simulink model "sschdlexSwissRectifierExample"  (R2023b)
settings: Solver=FixedStepDiscrete  StartTime=0.0  StopTime=.03  RelTol=1e-3  AbsTol=1e-3
InitFcn:
  | freqMain = 50;
  | Vrms=230;
  | Vin = Vrms * sqrt(2);
  | Vout=325;
  | freqSwitch=36e3;
  | PoutMax = 7.5e3;
  | loadPercent = 50;
  | RLoad = Vout^2/(PoutMax*(loadPercent/100));
  | COut = 470e-6;
  | LDC = 305e-6;
  | LF = 85e-6;
  | CF = 4.4e-6;
libraries: fl_lib x53, nesl_utility x20, ee_lib x8, simulink x2, slpidlib x2, powerlib_meascontrol x1
settings Model: DataTypeOverride=Off  Creator=The MathWorks, Inc.  LastModifiedBy=The MathWorks, Inc.
settings SolverCC: AutoScaleAbsTol=off  AlgebraicLoopSolver=TrustRegion
settings DataIOCC: LimitDataPoints=on  MaxDataPoints=10000  SaveOutput=off  SaveTime=off  ReturnWorkspaceOutputs=off
settings OptimizationCC: BlockReduction=off  ConditionallyExecuteInputs=off  DefaultParameterBehavior=Inlined  LifeSpan=inf
settings DebuggingCC: AlgebraicLoopMsg=error  SingleTaskRateTransMsg=error  UnconnectedInputMsg=warning  UnconnectedOutputMsg=warning  UnconnectedLineMsg=warning  AllowSymbolicDim=off  PregeneratedLibrarySubsystemCodeDiagnostic=none  SFUnexpectedBacktrackingDiag=warning  SFNoUnconditionalDefaultTransitionDiag=warning  SFExecutionAtInitializationDiag=none  ArithmeticOperatorsInVariantConditions=warning
settings HardwareCC: ProdBitPerPointer=32  ProdBitPerSizeT=32  ProdBitPerPtrDiffT=32  ProdLargestAtomicFloat=None  ProdIntDivRoundTo=Undefined  ProdEndianess=Unspecified  ProdWordSize=32  ProdHWDeviceType=ASIC/FPGA->ASIC/FPGA  TargetBitPerPointer=64  TargetBitPerSizeT=64  TargetBitPerPtrDiffT=64  TargetLongLongMode=on  TargetIntDivRoundTo=Zero  TargetEndianess=LittleEndian  TargetWordSize=64  TargetHWDeviceType=Custom Processor->MATLAB Host Computer  ProdEqTarget=off
settings ModelReferenceCC: EnableRefExpFcnMdlSchedulingChecks=on
settings SFSimCC: SimUseLocalCustomCode=off
settings RTWCC: RTWUseLocalCustomCode=off
settings CodeAppCC: StateflowObjectComments=on
settings GRTTargetCC: TargetLangStandard=C89/C90 (ANSI)
settings ConfigComp: CovMetricSettings=dw  CovSaveCumulativeToWorkspaceVar=on  CovSaveSingleToWorkspaceVar=on  CovExternalEMLEnable=off  CovSFcnEnable=off
settings SimscapeCC: SimscapeLogType=all  SimscapeLogDataHistory=10000

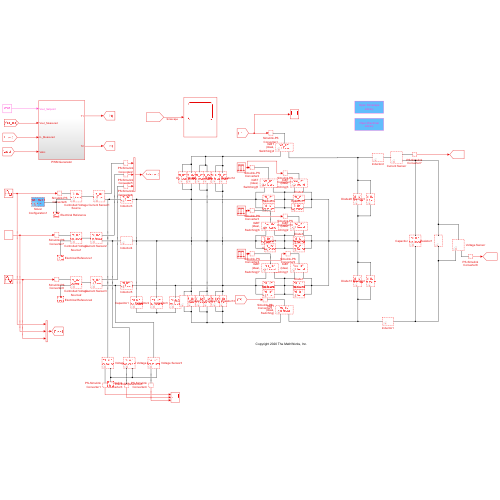
[thumbnail: Simulink's stored preview of the top-level diagram]
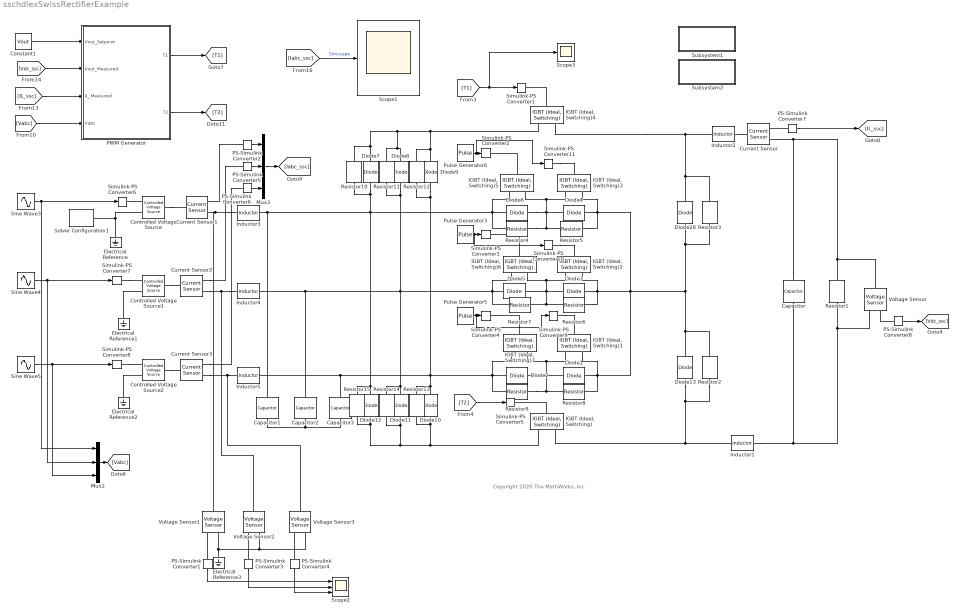
== system sschdlexSwissRectifierExample ==
  note: Copyright 2020 The MathWorks, Inc.
  Capacitor : fl_lib/Electrical/Electrical Elements/Capacitor  c=COut F  r=1e-6 Ohm  g=0 1/Ohm  i_specify=off  i_priority=None  i=0 A  i_nominal_specify=off  i_nominal_unit=A  i_nominal_value=1  v_specify=off  v_priority=None  v=0 V  v_nominal_specify=off  v_nominal_unit=V  v_nominal_value=1  vc_specify=off  vc_priority=High  vc=400 V  vc_nominal_specify=off  vc_nominal_unit=V  vc_nominal_value=1
  Capacitor1 : fl_lib/Electrical/Electrical Elements/Capacitor  c=CF F  r=1e-6 Ohm  g=0 1/Ohm  i_specify=off  i_priority=None  i=0 A  i_nominal_specify=off  i_nominal_unit=A  i_nominal_value=1  v_specify=off  v_priority=None  v=0 V  v_nominal_specify=off  v_nominal_unit=V  v_nominal_value=1  vc_specify=off  vc_priority=High  vc=0 V  vc_nominal_specify=off  vc_nominal_unit=V  vc_nominal_value=1
  Capacitor2 : fl_lib/Electrical/Electrical Elements/Capacitor  c=CF F  r=1e-6 Ohm  g=0 1/Ohm  i_specify=off  i_priority=None  i=0 A  i_nominal_specify=off  i_nominal_unit=A  i_nominal_value=1  v_specify=off  v_priority=None  v=0 V  v_nominal_specify=off  v_nominal_unit=V  v_nominal_value=1  vc_specify=off  vc_priority=High  vc=0 V  vc_nominal_specify=off  vc_nominal_unit=V  vc_nominal_value=1
  Capacitor3 : fl_lib/Electrical/Electrical Elements/Capacitor  c=CF F  r=1e-6 Ohm  g=0 1/Ohm  i_specify=off  i_priority=None  i=0 A  i_nominal_specify=off  i_nominal_unit=A  i_nominal_value=1  v_specify=off  v_priority=None  v=0 V  v_nominal_specify=off  v_nominal_unit=V  v_nominal_value=1  vc_specify=off  vc_priority=High  vc=0 V  vc_nominal_specify=off  vc_nominal_unit=V  vc_nominal_value=1
  Constant1 : Constant  Value=Vout
  Controlled Voltage Source : fl_lib/Electrical/Electrical Sources/Controlled Voltage Source
  Controlled Voltage Source1 : fl_lib/Electrical/Electrical Sources/Controlled Voltage Source
  Controlled Voltage Source2 : fl_lib/Electrical/Electrical Sources/Controlled Voltage Source
  Current Sensor{,1..3} (4 alike) : fl_lib/Electrical/Electrical Sensors/Current Sensor
  Diode{1..13,28} (14 alike) : fl_lib/Electrical/Electrical Elements/Diode  Vf=0.8 V  Ron=0.001 Ohm  Goff=1e-8 1/Ohm  i_specify=on  i_priority=High  i=0 A  i_nominal_specify=off  i_nominal_unit=A  i_nominal_value=1  v_specify=off  v_priority=None  v=0 V  v_nominal_specify=off  v_nominal_unit=V  v_nominal_value=1
  Electrical Reference{,1..3} (4 alike) : fl_lib/Electrical/Electrical Elements/Electrical Reference
  IGBT (Ideal, Switching){,1..7} (8 alike) : ee_lib/Semiconductors & Converters/IGBT (Ideal, Switching)  Vf=0.8 V  Ron=0.001 Ohm  Goff=1e-5 1/Ohm  Vth=.5 V  diode_param=1  diode_Vf=0.8 V  diode_Ron=0.001 Ohm  diode_Goff=1e-5 1/Ohm  diode_C=50e-9 F  diode_iRM=-235 A  diode_iF=300 A  diode_idot=-50 A/us  diode_trr_param=1  diode_trr_factor=3  diode_trr=15 us  diode_Qrr=1500 s*uA  thermal_loss_option=2  Von_data=[0, 1.1, 1.3, 1.45, 1.75, 2.25, 2.7; 0, 1, 1.15, 1.35, 1.7, 2.35, 3] V  Eon_data=[0, .29, 1.43, 2.86, 5.71, 13.14, 22.86; 0, .57, 2.63, 5.14, 10.29, 20.57, 30.29] * 1e-3 J  Eoff_data=[0, .21, 1.07, 2.14, 4.29, 9.86, 17.14; 0, .43, 1.97, 3.86, 7.71, 15.43, 22.71] * 1e-3 J  Tj=[298.15, 398.15] K  Iout_data=[0, 10, 50, 100, 200, 400, 600] A  Eon_scalar=22.86e-3 J  Eoff_scalar=17.14e-3 J  Voff=300 V  Iout_scalar=600 A  diodeModelType=ee.enum.converters.diodeModelType.pwl  diode_IfMat=[.07, .12, .19, 1.75, 4.24, 7.32, 11.2; .16, .3, .72, 2.14, 4.02, 6.35, 9.12] A  diode_TjVec=[25, 125] degC  diode_VfVec=[.5, .7, .9, 1.3, 1.7, 2.1, 2.5] V  thermal_network_parameterization=ee.enum.thermalNetworkTopology.external  Rth=[.08, .5] K/W  Rth_Foster=[.08, .14, .22, .16] K/W  thermal_mass_parameterization=ee.enum.thermalNetwork.timeconstant  thermal_mass=[.01, .5] J/K  thermal_mass_Foster=[.001, .005, .05, .5] J/K  thermal_time_constant=[.001, .2] s  thermal_time_constant_Foster=[7e-05, .0007, .01, .08] s  thermal_mass_initial_temperatures=[25, 25] degC  junction_thermal_mass=0.01 J/K  vT_specify=off  vT_priority=None  vT=0 V  vT_nominal_specify=off  vT_nominal_unit=V  vT_nominal_value=1  Qj_specify=off  Qj_priority=None  Qj=0 W  Qj_nominal_specify=off  Qj_nominal_unit=W  Qj_nominal_value=1  junction_temperature_specify=off  junction_temperature_priority=None  junction_temperature=25 degC  junction_temperature_nominal_specify=off  junction_temperature_nominal_unit=degC  junction_temperature_nominal_value=1  temperatureStepFromSwitchLoss_specify=off  temperatureStepFromSwitchLoss_priority=None  temperatureStepFromSwitchLoss=0 K
  Inductor1 : fl_lib/Electrical/Electrical Elements/Inductor  l=LDC H  r=0 Ohm  g=1e-9 1/Ohm  i_specify=off  i_priority=None  i=0 A  i_nominal_specify=off  i_nominal_unit=A  i_nominal_value=1  v_specify=off  v_priority=None  v=0 V  v_nominal_specify=off  v_nominal_unit=V  v_nominal_value=1  i_L_specify=off  i_L_priority=High  i_L=0 A  i_L_nominal_specify=off  i_L_nominal_unit=A  i_L_nominal_value=1
  Inductor2 : fl_lib/Electrical/Electrical Elements/Inductor  l=LDC H  r=0 Ohm  g=1e-9 1/Ohm  i_specify=off  i_priority=None  i=0 A  i_nominal_specify=off  i_nominal_unit=A  i_nominal_value=1  v_specify=off  v_priority=None  v=0 V  v_nominal_specify=off  v_nominal_unit=V  v_nominal_value=1  i_L_specify=off  i_L_priority=High  i_L=0 A  i_L_nominal_specify=off  i_L_nominal_unit=A  i_L_nominal_value=1
  Inductor3 : fl_lib/Electrical/Electrical Elements/Inductor  l=LF H  r=0 Ohm  g=1e-9 1/Ohm  i_specify=off  i_priority=None  i=0 A  i_nominal_specify=off  i_nominal_unit=A  i_nominal_value=1  v_specify=off  v_priority=None  v=0 V  v_nominal_specify=off  v_nominal_unit=V  v_nominal_value=1  i_L_specify=off  i_L_priority=High  i_L=0 A  i_L_nominal_specify=off  i_L_nominal_unit=A  i_L_nominal_value=1
  Inductor4 : fl_lib/Electrical/Electrical Elements/Inductor  l=LF H  r=0 Ohm  g=1e-9 1/Ohm  i_specify=off  i_priority=None  i=0 A  i_nominal_specify=off  i_nominal_unit=A  i_nominal_value=1  v_specify=off  v_priority=None  v=0 V  v_nominal_specify=off  v_nominal_unit=V  v_nominal_value=1  i_L_specify=off  i_L_priority=High  i_L=0 A  i_L_nominal_specify=off  i_L_nominal_unit=A  i_L_nominal_value=1
  Inductor5 : fl_lib/Electrical/Electrical Elements/Inductor  l=LF H  r=0 Ohm  g=1e-9 1/Ohm  i_specify=off  i_priority=None  i=0 A  i_nominal_specify=off  i_nominal_unit=A  i_nominal_value=1  v_specify=off  v_priority=None  v=0 V  v_nominal_specify=off  v_nominal_unit=V  v_nominal_value=1  i_L_specify=off  i_L_priority=High  i_L=0 A  i_L_nominal_specify=off  i_L_nominal_unit=A  i_L_nominal_value=1
  Mux2 : Mux  Inputs=3
  Mux3 : Mux  Inputs=3
  PS-Simulink Converter{1..8} (8 alike) : nesl_utility/PS-Simulink Converter  PhysicalDomain=network_engine_domain  SubClassName=ps_output  LeftPortType=input  RightPortType=output  PseudoPeriodic=off  Frequencies=[]  Unit=1  AffineConversion=off
  PWM Generator : Subsystem
  Pulse Generator3 : DiscretePulseGenerator  Period=freqSwitch*100/(2*freqMain)  PulseWidth=freqSwitch*100/(2*freqMain)/3  PhaseDelay=freqSwitch*100*(2/3-1/6)*1/(2*freqMain)  SampleTime=1/freqSwitch/100
  Pulse Generator5 : DiscretePulseGenerator  Period=freqSwitch*100/(2*freqMain)  PulseWidth=freqSwitch*100/(2*freqMain)/3  PhaseDelay=round((1/3-1/6)*1/(2*freqMain)*freqSwitch*100)  SampleTime=1/freqSwitch/100
  Pulse Generator6 : DiscretePulseGenerator  Period=freqSwitch*100/(2*freqMain)  PulseWidth=freqSwitch*100/(2*freqMain)/3  PhaseDelay=freqSwitch*100*(0/3-1/6)*1/(2*freqMain)  SampleTime=1/freqSwitch/100
  Resistor1 : fl_lib/Electrical/Electrical Elements/Resistor  R=RLoad Ohm  i_specify=off  i_priority=None  i=0 A  i_nominal_specify=off  i_nominal_unit=A  i_nominal_value=1  v_specify=off  v_priority=None  v=0 V  v_nominal_specify=off  v_nominal_unit=V  v_nominal_value=1
  Resistor{2..15} (14 alike) : fl_lib/Electrical/Electrical Elements/Resistor  R=500 Ohm  i_specify=off  i_priority=None  i=0 A  i_nominal_specify=off  i_nominal_unit=A  i_nominal_value=1  v_specify=off  v_priority=None  v=0 V  v_nominal_specify=off  v_nominal_unit=V  v_nominal_value=1
  Scope1 : Scope
  Scope2 : Scope  NumInputPorts=3
  Scope3 : Scope
  Simulink-PS Converter{1..11} (11 alike) : nesl_utility/Simulink-PS Converter  PhysicalDomain=network_engine_domain  SubClassName=ps_input  LeftPortType=input  RightPortType=output  PseudoPeriodic=off  Frequencies=[]  NoiseDistribution=none  NoiseParameters=[]  Unit=1  AffineConversion=off  FilteringAndDerivatives=provide  SimscapeFilterOrder=1  InputFilterTimeConstant=0.001  UdotUserProvided=0
  Sine Wave3 : Sin  Amplitude=Vin  Frequency=freqMain*2*pi  SampleTime=1/freqSwitch/100
  Sine Wave4 : Sin  Amplitude=Vin  Frequency=freqMain*2*pi  Phase=-120*pi/180  SampleTime=1/freqSwitch/100
  Sine Wave5 : Sin  Amplitude=Vin  Frequency=freqMain*2*pi  Phase=120*pi/180  SampleTime=1/freqSwitch/100
  Solver Configuration1 : nesl_utility/Solver Configuration  PhysicalDomain=network_engine_domain  SubClassName=solver  LeftPortType=input  RightPortType=generic  Tones=[]  Harmonics=[]  SimulateNoise=off  Profile=off  UseLocalSampling=off  EnableSwitchedLinearOptims=on  FrequencyDomain=off  UseCCode=off  RelTol=0.001  AbsTol=1e-06  MinStep=1e-09  ToWorkspace=off  RevertToSquareIcSolve=off  NumHomotopyIterations=100  PhasorMode=off  PhasorModeNumHarmonics=1  DoDC=off  ResidualTolerance=1e-09  UseLocalSolver=on  LocalSolverChoice=NE_BACKWARD_EULER_ADVANCER  LocalSolverSampleTime=1/freqSwitch/100  DoFixedCost=off  MaxNonlinIter=3  MaxModeIter=2  LinearAlgebra=auto  EquationFormulation=NE_TIME_EF  DelaysMemoryBudget=1024  AutomaticFiltering=off  FilteringTimeConstant=0.001  PartitionStorageMethod=AS_NEEDED  PartitionMemoryBudget=1024  PartitionMethod=FAST
  Subsystem1 : Subsystem
      settings: OpenFcn=open_system('simscape')
      mask Display: disp(sprintf('Open Simscape\nLibrary'));
  Subsystem2 : Subsystem
      settings: OpenFcn=|
      | load_system('fl_lib');
      | open_system('fl_lib/Electrical');
      mask Display: disp(sprintf('Open Electrical\nLibrary'));
  Voltage Sensor{,1..3} (4 alike) : fl_lib/Electrical/Electrical Sensors/Voltage Sensor
  wires:
  [T1] -> Scope3/1, Simulink-PS Converter1/1
  PWM Generator/1(T1) -> [T1]
  Pulse Generator5/1 -> Simulink-PS Converter9/1, Simulink-PS Converter4/1
  PS-Simulink Converter7/1 -> [IL_ssc]
  Sine Wave5/1 -> Mux2/3, Simulink-PS Converter8/1
  Sine Wave3/1 -> Mux2/1, Simulink-PS Converter6/1
  [Vabc] -> PWM Generator/4(Vabc)
  Sine Wave4/1 -> Mux2/2, Simulink-PS Converter7/1
  PS-Simulink Converter3/1 -> Scope2/2
  PWM Generator/2(T2) -> [T2]
  PS-Simulink Converter2/1 -> Mux3/1
  [IL_ssc] -> PWM Generator/3(IL_Measured)
  Pulse Generator3/1 -> Simulink-PS Converter10/1, Simulink-PS Converter3/1
  [Iabc_ssc] -> Scope1/1  "Simscape"
  Constant1/1 -> PWM Generator/1(Vout_Setpoint)
  [T2] -> Simulink-PS Converter5/1
  Mux2/1 -> [Vabc]
  PS-Simulink Converter5/1 -> Mux3/2
  [Vdc_ssc] -> PWM Generator/2(Vout_Measured)
  PS-Simulink Converter1/1 -> Scope2/1
  Pulse Generator6/1 -> Simulink-PS Converter11/1, Simulink-PS Converter2/1
  PS-Simulink Converter4/1 -> Scope2/3
  PS-Simulink Converter6/1 -> Mux3/3
  PS-Simulink Converter8/1 -> [Vdc_ssc]
  Mux3/1 -> [Iabc_ssc]
  connections:
  Diode12/LConn1 -- "IGBT (Ideal, Switching)"/RConn2 -- Resistor13/LConn1 -- Diode10/LConn1 -- Resistor14/LConn1 -- Diode11/LConn1 -- Resistor15/LConn1
  Diode28/LConn1 -- "IGBT (Ideal, Switching)3"/RConn1 -- Resistor5/LConn1 -- Diode4/RConn1 -- "IGBT (Ideal, Switching)1"/RConn1 -- Resistor8/LConn1 -- Diode1/RConn1 -- "IGBT (Ideal, Switching)2"/RConn1 -- Resistor6/LConn1 -- Diode3/RConn1 -- Resistor2/LConn1 -- Diode13/RConn1 -- Resistor3/RConn1
  Diode7/LConn1 -- "IGBT (Ideal, Switching)5"/RConn1 -- Resistor4/RConn1 -- Diode6/RConn1 -- Inductor3/RConn1 -- Capacitor1/LConn1 -- Resistor15/RConn1 -- Diode12/RConn1 -- Resistor10/LConn1
  "IGBT (Ideal, Switching)6"/RConn1 -- Resistor7/RConn1 -- Diode5/RConn1 -- Diode8/LConn1 -- Resistor11/LConn1 -- Capacitor2/LConn1 -- Inductor4/RConn1 -- Resistor14/RConn1 -- Diode11/RConn1
  Solver Configuration1/RConn1 -- Electrical Reference/LConn1 -- Controlled Voltage Source/RConn2
  Voltage Sensor2/RConn2 -- Electrical Reference3/LConn1 -- Voltage Sensor1/RConn2 -- Voltage Sensor3/RConn2
  Inductor1/LConn1 -- "IGBT (Ideal, Switching)"/RConn1 -- Resistor2/RConn1 -- Diode13/LConn1
  "IGBT (Ideal, Switching)1"/RConn2 -- "IGBT (Ideal, Switching)7"/RConn2 -- Resistor9/LConn1 -- Resistor8/RConn1 -- Diode1/LConn1 -- Diode2/LConn1
  Diode7/RConn1 -- "IGBT (Ideal, Switching)4"/RConn1 -- Resistor12/RConn1 -- Diode9/RConn1 -- Diode8/RConn1 -- Resistor11/RConn1 -- Resistor10/RConn1
  "IGBT (Ideal, Switching)6"/LConn1 -- Simulink-PS Converter3/RConn1
  Capacitor/LConn1 -- Current Sensor/RConn2 -- Resistor1/LConn1 -- Voltage Sensor/LConn1
  "IGBT (Ideal, Switching)7"/LConn1 -- Simulink-PS Converter4/RConn1
  Diode3/LConn1 -- Resistor6/RConn1 -- Resistor7/LConn1 -- Diode5/LConn1 -- "IGBT (Ideal, Switching)2"/RConn2 -- "IGBT (Ideal, Switching)6"/RConn2
  "IGBT (Ideal, Switching)3"/RConn2 -- "IGBT (Ideal, Switching)5"/RConn2 -- Resistor5/RConn1 -- Resistor4/LConn1 -- Diode4/LConn1 -- Diode6/LConn1
  Diode28/RConn1 -- "IGBT (Ideal, Switching)4"/RConn2 -- Inductor2/LConn1 -- Resistor3/LConn1
  "IGBT (Ideal, Switching)5"/LConn1 -- Simulink-PS Converter2/RConn1
  Resistor1/RConn1 -- Capacitor/RConn1 -- Inductor1/RConn1 -- Voltage Sensor/RConn2
  Diode9/LConn1 -- "IGBT (Ideal, Switching)7"/RConn1 -- Resistor9/RConn1 -- Diode2/RConn1 -- Inductor5/RConn1 -- Capacitor3/LConn1 -- Resistor13/RConn1 -- Diode10/RConn1 -- Resistor12/LConn1
  Capacitor3/RConn1 -- Capacitor1/RConn1 -- Capacitor2/RConn1
  Inductor5/LConn1 -- Voltage Sensor3/LConn1 -- Current Sensor3/RConn2
  Inductor4/LConn1 -- Voltage Sensor2/LConn1 -- Current Sensor2/RConn2
  Inductor3/LConn1 -- Current Sensor1/RConn2 -- Voltage Sensor1/LConn1
  Current Sensor3/RConn1 -- PS-Simulink Converter6/LConn1
  "IGBT (Ideal, Switching)4"/LConn1 -- Simulink-PS Converter1/RConn1
  Simulink-PS Converter7/RConn1 -- Controlled Voltage Source1/RConn1
  PS-Simulink Converter8/LConn1 -- Voltage Sensor/RConn1
  Current Sensor2/RConn1 -- PS-Simulink Converter5/LConn1
  Simulink-PS Converter8/RConn1 -- Controlled Voltage Source2/RConn1
  PS-Simulink Converter3/LConn1 -- Voltage Sensor2/RConn1
  Electrical Reference1/LConn1 -- Controlled Voltage Source1/RConn2
  Inductor2/RConn1 -- Current Sensor/LConn1
  PS-Simulink Converter1/LConn1 -- Voltage Sensor1/RConn1
  "IGBT (Ideal, Switching)"/LConn1 -- Simulink-PS Converter5/RConn1
  PS-Simulink Converter7/LConn1 -- Current Sensor/RConn1
  PS-Simulink Converter4/LConn1 -- Voltage Sensor3/RConn1
  PS-Simulink Converter2/LConn1 -- Current Sensor1/RConn1
  Electrical Reference2/LConn1 -- Controlled Voltage Source2/RConn2
  Controlled Voltage Source/LConn1 -- Current Sensor1/LConn1
  Simulink-PS Converter6/RConn1 -- Controlled Voltage Source/RConn1
  Controlled Voltage Source1/LConn1 -- Current Sensor2/LConn1
  Controlled Voltage Source2/LConn1 -- Current Sensor3/LConn1
  Simulink-PS Converter11/RConn1 -- "IGBT (Ideal, Switching)3"/LConn1
  Simulink-PS Converter10/RConn1 -- "IGBT (Ideal, Switching)2"/LConn1
  Simulink-PS Converter9/RConn1 -- "IGBT (Ideal, Switching)1"/LConn1

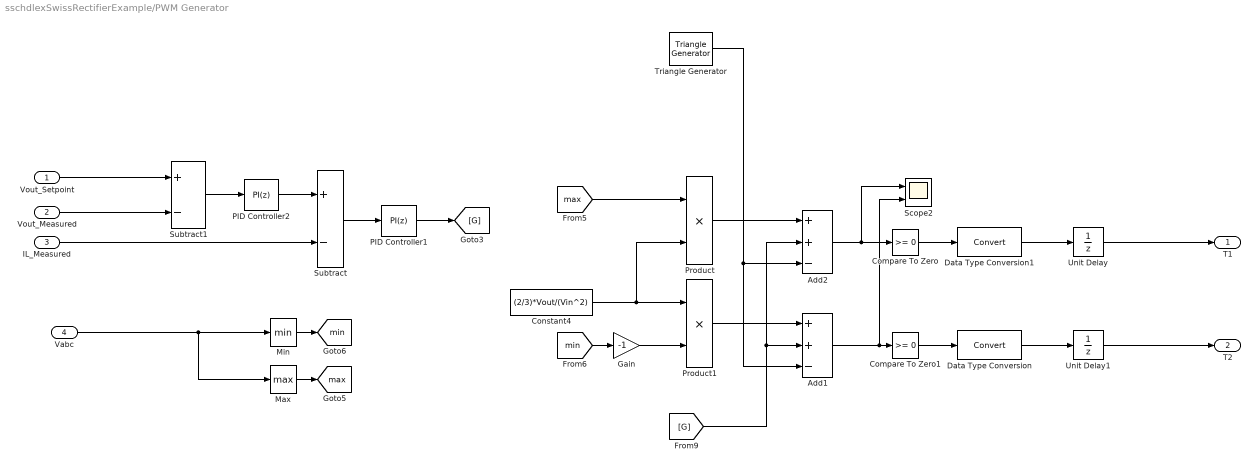
== system sschdlexSwissRectifierExample/PWM Generator ==
  Vout_Setpoint : Inport
  Vout_Measured : Inport  Port=2
  IL_Measured : Inport  Port=3
  Vabc : Inport  Port=4
  Add1 : Sum  Inputs=++-
  Add2 : Sum  Inputs=++-
  Compare To Zero : simulink/Logic and Bit Operations/Compare To Zero  relop=>=  OutDataTypeStr=boolean
  Compare To Zero1 : simulink/Logic and Bit Operations/Compare To Zero  relop=>=  OutDataTypeStr=boolean
  Constant4 : Constant  Value=(2/3)*Vout/(Vin^2)
  Data Type Conversion : DataTypeConversion  SaturateOnIntegerOverflow=off  RndMeth=Floor
  Data Type Conversion1 : DataTypeConversion  SaturateOnIntegerOverflow=off  RndMeth=Floor
  Gain : Gain  Gain=-1
  Max : MinMax  Function=max
  Min : MinMax
  PID Controller1 : slpidlib/PID Controller  Controller=PI  Form=Parallel  TimeDomain=Discrete-time  UseExternalTs=off  SampleTime=-1  IntegratorMethod=Forward Euler  FilterMethod=Forward Euler  ControllerParametersSource=internal  P=0.1  I=10000/5  UseKiTs=off  D=0  N=100  UseFilter=on  TunerSelectOption=Transfer Function Based (PID Tuner App)  InitialConditionSource=internal  InitialConditionForIntegrator=0  InitialConditionForFilter=0  DifferentiatorICPrevScaledInput=0  ExternalReset=none  TrackingMode=off  Kt=1  LimitOutput=off  SatLimitsSource=internal  UpperSaturationLimit=inf  LowerSaturationLimit=-inf  LinearizeAsGain=on  AntiWindupMode=none  Kb=1  LimitIntegrator=off  UpperIntegratorSaturationLimit=inf  LowerIntegratorSaturationLimit=-inf  POutMin=[]  POutMax=[]  IOutMin=[]  IOutMax=[]  DOutMin=[]  DOutMax=[]  NOutMin=[]  NOutMax=[]  SumOutMin=[]  SumOutMax=[]  SaturationOutMin=[]  SaturationOutMax=[]  PParamMin=[]  PParamMax=[]  IParamMin=[]  IParamMax=[]  DParamMin=[]  DParamMax=[]  NParamMin=[]  NParamMax=[]  KbParamMin=[]  KbParamMax=[]  KtParamMin=[]  KtParamMax=[]  KbOutMin=[]  KbOutMax=[]  KtOutMin=[]  KtOutMax=[]  IntegratorOutMin=[]  IntegratorOutMax=[]  FilterOutMin=[]  FilterOutMax=[]  SumI1OutMin=[]  SumI1OutMax=[]  SumI2OutMin=[]  SumI2OutMax=[]  SumI3OutMin=[]  SumI3OutMax=[]  SumI4OutMin=[]  SumI4OutMax=[]  SumDOutMin=[]  SumDOutMax=[]  DifferentiatorOutMin=[]  DifferentiatorOutMax=[]  FilterDiffOutCoefMin=[]  FilterDiffOutCoefMax=[]  ReciprocalOutMin=[]  ReciprocalOutMax=[]  SumDenOutMin=[]  SumDenOutMax=[]  SumNumOutMin=[]  SumNumOutMax=[]  DivideOutMin=[]  DivideOutMax=[]  UdiffTsProdOutMin=[]  UdiffTsProdOutMax=[]  NTsProdOutMin=[]  NTsProdOutMax=[]  UintegralTsProdOutMin=[]  UintegralTsProdOutMax=[]  UngainTsProdOutMin=[]  UngainTsProdOutMax=[]  ClampingZeroOutDataTypeStr=Inherit: Inherit via back propagation  ClampingZeroOutMin=[]  ClampingZeroOutMax=[]  FilterDenConstantOutDataTypeStr=Inherit: Inherit via back propagation  FilterDenConstantOutMin=[]  FilterDenConstantOutMax=[]  PCopyOutDataTypeStr=Inherit: Inherit via back propagation  PCopyOutMin=[]  PCopyOutMax=[]  NCopyOutDataTypeStr=Inherit: Inherit via back propagation  NCopyOutMin=[]  NCopyOutMax=[]  IntegratorContinuousStateAttributes=''  IntegratorStateMustResolveToSignalObject=off  IntegratorRTWStateStorageClass=Auto  FilterContinuousStateAttributes=''  FilterStateMustResolveToSignalObject=off  FilterRTWStateStorageClass=Auto  ParallelPVariant=InternalParameters  IdealPVariant=Disabled  IVariant=InternalParameters  DVariant=Disabled  IntegratorVariant=Discrete  SatVariant=Disabled  AWVariant=Passthrough  PCopyVariant=Disabled  TRVariant=Disabled  FdbkBlocksVariant=Forward  IdealPFdbkVariant=Disabled  SatFdbkVariant=Disabled  DerivativeFilterVariant=Disabled  NVariant=Disabled  NCopyVariant=Disabled_SignalSpec  FilterICVariant=Disabled  IntegratorICVariant=InternalICs  ExternalResetVariant=Disabled  TRSumVariant=Passthrough  SumFdbkVariant=Disabled  SumVariant=Sum_PI  TsampFilterVariant=InternalTs  TsampNgainVariant=Passthrough  TsampIntegralVariant=Disabled_SignalSpec  ExternalSaturationOutDataTypeStr=Inherit: Same as second input
  PID Controller2 : slpidlib/PID Controller  Controller=PI  Form=Parallel  TimeDomain=Discrete-time  UseExternalTs=off  SampleTime=-1  IntegratorMethod=Forward Euler  FilterMethod=Forward Euler  ControllerParametersSource=internal  P=1/10  I=10  UseKiTs=off  D=0  N=100  UseFilter=on  TunerSelectOption=Transfer Function Based (PID Tuner App)  InitialConditionSource=internal  InitialConditionForIntegrator=0  InitialConditionForFilter=0  DifferentiatorICPrevScaledInput=0  ExternalReset=none  TrackingMode=off  Kt=1  LimitOutput=off  SatLimitsSource=internal  UpperSaturationLimit=inf  LowerSaturationLimit=-inf  LinearizeAsGain=on  AntiWindupMode=none  Kb=1  LimitIntegrator=off  UpperIntegratorSaturationLimit=inf  LowerIntegratorSaturationLimit=-inf  POutMin=[]  POutMax=[]  IOutMin=[]  IOutMax=[]  DOutMin=[]  DOutMax=[]  NOutMin=[]  NOutMax=[]  SumOutMin=[]  SumOutMax=[]  SaturationOutMin=[]  SaturationOutMax=[]  PParamMin=[]  PParamMax=[]  IParamMin=[]  IParamMax=[]  DParamMin=[]  DParamMax=[]  NParamMin=[]  NParamMax=[]  KbParamMin=[]  KbParamMax=[]  KtParamMin=[]  KtParamMax=[]  KbOutMin=[]  KbOutMax=[]  KtOutMin=[]  KtOutMax=[]  IntegratorOutMin=[]  IntegratorOutMax=[]  FilterOutMin=[]  FilterOutMax=[]  SumI1OutMin=[]  SumI1OutMax=[]  SumI2OutMin=[]  SumI2OutMax=[]  SumI3OutMin=[]  SumI3OutMax=[]  SumI4OutMin=[]  SumI4OutMax=[]  SumDOutMin=[]  SumDOutMax=[]  DifferentiatorOutMin=[]  DifferentiatorOutMax=[]  FilterDiffOutCoefMin=[]  FilterDiffOutCoefMax=[]  ReciprocalOutMin=[]  ReciprocalOutMax=[]  SumDenOutMin=[]  SumDenOutMax=[]  SumNumOutMin=[]  SumNumOutMax=[]  DivideOutMin=[]  DivideOutMax=[]  UdiffTsProdOutMin=[]  UdiffTsProdOutMax=[]  NTsProdOutMin=[]  NTsProdOutMax=[]  UintegralTsProdOutMin=[]  UintegralTsProdOutMax=[]  UngainTsProdOutMin=[]  UngainTsProdOutMax=[]  ClampingZeroOutDataTypeStr=Inherit: Inherit via back propagation  ClampingZeroOutMin=[]  ClampingZeroOutMax=[]  FilterDenConstantOutDataTypeStr=Inherit: Inherit via back propagation  FilterDenConstantOutMin=[]  FilterDenConstantOutMax=[]  PCopyOutDataTypeStr=Inherit: Inherit via back propagation  PCopyOutMin=[]  PCopyOutMax=[]  NCopyOutDataTypeStr=Inherit: Inherit via back propagation  NCopyOutMin=[]  NCopyOutMax=[]  IntegratorContinuousStateAttributes=''  IntegratorStateMustResolveToSignalObject=off  IntegratorRTWStateStorageClass=Auto  FilterContinuousStateAttributes=''  FilterStateMustResolveToSignalObject=off  FilterRTWStateStorageClass=Auto  ParallelPVariant=InternalParameters  IdealPVariant=Disabled  IVariant=InternalParameters  DVariant=Disabled  IntegratorVariant=Discrete  SatVariant=Disabled  AWVariant=Passthrough  PCopyVariant=Disabled  TRVariant=Disabled  FdbkBlocksVariant=Forward  IdealPFdbkVariant=Disabled  SatFdbkVariant=Disabled  DerivativeFilterVariant=Disabled  NVariant=Disabled  NCopyVariant=Disabled_SignalSpec  FilterICVariant=Disabled  IntegratorICVariant=InternalICs  ExternalResetVariant=Disabled  TRSumVariant=Passthrough  SumFdbkVariant=Disabled  SumVariant=Sum_PI  TsampFilterVariant=InternalTs  TsampNgainVariant=Passthrough  TsampIntegralVariant=Disabled_SignalSpec  ExternalSaturationOutDataTypeStr=Inherit: Same as second input
  Product : Product
  Product1 : Product
  Scope2 : Scope  NumInputPorts=2
  Subtract : Sum  Inputs=+-
  Subtract1 : Sum  Inputs=+-
  Triangle Generator : powerlib_meascontrol/Pulse & Signal Generators/Triangle Generator  Freq=freqSwitch  Phase=0  Ts=1/freqSwitch/100
  Unit Delay : UnitDelay  SampleTime=-1  HasFrameUpgradeWarning=on
  Unit Delay1 : UnitDelay  SampleTime=-1  HasFrameUpgradeWarning=on
  T1 : Outport  VectorParamsAs1DForOutWhenUnconnected=off
  T2 : Outport  Port=2  VectorParamsAs1DForOutWhenUnconnected=off
  tag scope: max=global, min=global
  wires:
  Vabc/1 -> Max/1, Min/1
  Constant4/1 -> Product/2, Product1/1
  Compare To Zero1/1 -> Data Type Conversion/1
  [G] -> Add2/2, Add1/2
  Unit Delay1/1 -> T2/1
  IL_Measured/1 -> Subtract/2
  PID Controller2/1 -> Subtract/1
  Compare To Zero/1 -> Data Type Conversion1/1
  Add1/1 -> Compare To Zero1/1, Scope2/2
  Add2/1 -> Compare To Zero/1, Scope2/1
  Product/1 -> Add2/1
  Data Type Conversion1/1 -> Unit Delay/1
  Triangle Generator/1 -> Add2/3, Add1/3
  [max] -> Product/1
  Subtract/1 -> PID Controller1/1
  Product1/1 -> Add1/1
  Data Type Conversion/1 -> Unit Delay1/1
  Gain/1 -> Product1/2
  Max/1 -> [max]
  Min/1 -> [min]
  Subtract1/1 -> PID Controller2/1
  [min] -> Gain/1
  PID Controller1/1 -> [G]
  Vout_Measured/1 -> Subtract1/2
  Vout_Setpoint/1 -> Subtract1/1
  Unit Delay/1 -> T1/1

== system sschdlexSwissRectifierExample/Subsystem1 ==

== system sschdlexSwissRectifierExample/Subsystem2 ==
